simulink library "speedgoatlib_evse"  (R2024b)
settings: Solver=VariableStepAuto  StartTime=0.0  StopTime=10.0  RelTol=1e-3
undefined symbols (not defined in the file): sg_ev_charging_read_m, sg_ev_charging_write_m, sg_ev_isolation_read_m, sg_ev_parameter_read_m, sg_ev_parameter_write_m, sg_ev_precharge_read_m, sg_ev_precharge_write_m, sg_ev_status_m, sg_ev_stop_read_m, sg_ev_stop_write_m, sg_ev_welding_read_m, sg_ev_welding_write_m, sg_evse_charging_read_m, sg_evse_charging_write_m, sg_evse_isolation_read_m, sg_evse_isolation_write_m, sg_evse_parameter_read_m, sg_evse_parameter_write_m, sg_evse_precharge_read_m, sg_evse_precharge_write_m, sg_evse_status_m, sg_evse_stop_read_m, sg_evse_stop_write_m, sg_evse_welding_read_m, sg_evse_welding_write_m
libraries: speedgoatlib_mqtt x199, simulink x39, $bdroot x24
(part 3 of 8)

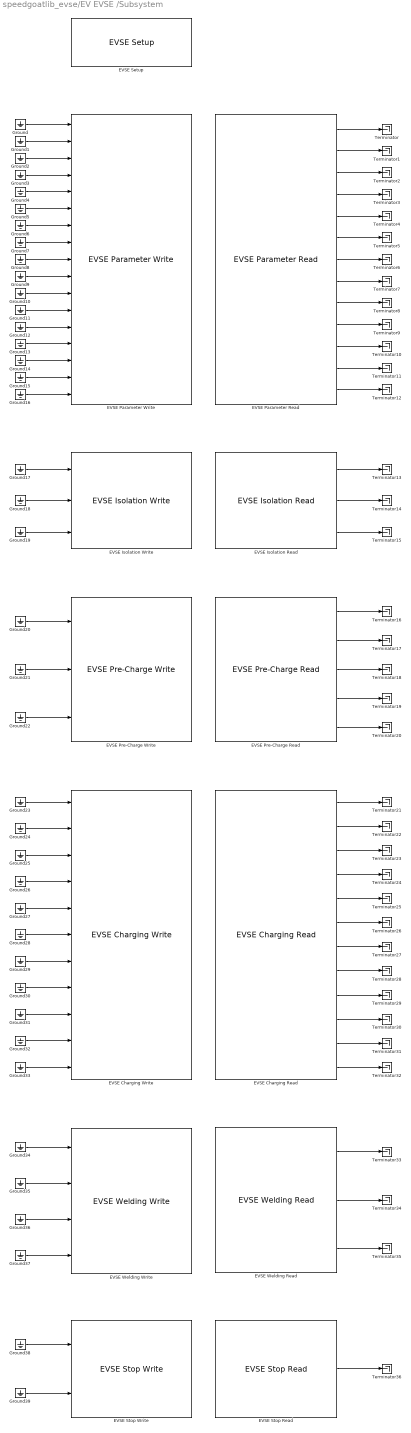
== system speedgoatlib_evse/EV EVSE /Subsystem ==
  "EVSE Charging Read " : $bdroot/Blocks by Charge State/EVSE Charging Read   parClientId=0  parConnectionId=0  parSampleTime=-1
  "EVSE Charging Write " : $bdroot/Blocks by Charge State/EVSE Charging Write   parClientId=0  parConnectionId=0  parSampleTime=-1  parEnNotification=off  parEnIsolationStatus=off  parEnStatusCode=off  parEnPresentVoltage=off  parEnPresentCurrent=off  parEnCurrentLimitAchieved=off  parEnVoltageLimitAchieved=off  parEnPowerLimitAchieved=off  parEnMaxVoltageLimit=off  parEnMaxCurrentLimit=off  parEnMaxPowerLimit=off
  "EVSE Isolation Read " : $bdroot/Blocks by Charge State/EVSE Isolation Read   parClientId=0  parConnectionId=0  parSampleTime=-1
  "EVSE Isolation Write " : $bdroot/Blocks by Charge State/EVSE Isolation Write   parClientId=0  parConnectionId=0  parSampleTime=-1  parEnEvseProcessing=off  parEnIsolationStatus=off  parEnStatusCode=off
  "EVSE Parameter Read " : $bdroot/Blocks by Charge State/EVSE Parameter Read   parClientId=0  parConnectionId=0  parSampleTime=-1
  "EVSE Parameter Write " : $bdroot/Blocks by Charge State/EVSE Parameter Write   parClientId=0  parConnectionId=0  parSampleTime=-1  parEnEvseProcessing=off  parEnSaScheduleList=off  parEnMaxVoltageLimit=off  parEnMaxCurrentLimit=off  parEnMaxPowerLimit=off  parEnMinVoltageLimit=off  parEnMinCurrentLimit=off  parEnCurrRegTol=off  parEnPeakCurrentRipple=off  parEnEnergyToBeDelivered=off  parEnNotificationMaxDelay=off  parEnNotification=off  parEnIsolationStatus=off  parEnStatusCode=off
  "EVSE Pre-Charge Read " : $bdroot/Blocks by Charge State/EVSE Pre-Charge Read   parClientId=0  parConnectionId=0  parSampleTime=-1
  "EVSE Pre-Charge Write " : $bdroot/Blocks by Charge State/EVSE Pre-Charge Write   parClientId=0  parConnectionId=0  parSampleTime=-1  parEnIsolationStatus=off  parEnStatusCode=off  parEnPresentVoltage=off
  "EVSE Setup " : $bdroot/Blocks by Charge State/EVSE Setup   parClientId=0  parConnectionId=0  parClientIdentifier='speedgoat'  parIpAddrStr='192.168.10.7'  parSampleTime=-1  parTcpPort=1883  parRemoteIpAddrStr='192.168.10.8'  parMaxVoltageLimit=480  parMaxCurrentLimit=100  parMinCurrentLimit=0  parMaxPowerLimit=60000  parMinVoltageLimit=12  parCurrRegTol=5  parPeakCurrentRipple=0
  "EVSE Stop Read " : $bdroot/Blocks by Charge State/EVSE Stop Read   parClientId=0  parConnectionId=0  parSampleTime=-1
  "EVSE Stop Write " : $bdroot/Blocks by Charge State/EVSE Stop Write   parClientId=0  parConnectionId=0  parSampleTime=-1  parEnStopProgress=off  parEnEvseProcessing=off
  "EVSE Welding Read " : $bdroot/Blocks by Charge State/EVSE Welding Read   parClientId=0  parConnectionId=0  parSampleTime=-1
  "EVSE Welding Write " : $bdroot/Blocks by Charge State/EVSE Welding Write   parClientId=0  parConnectionId=0  parSampleTime=-1  parEnNotification=off  parEnIsolationStatus=off  parEnStatusCode=off  parEnPresentVoltage=off
  Ground{,1..39} (40 alike) : Ground
  Terminator{,1..36} (37 alike) : Terminator
  wires:
  "EVSE Pre-Charge Read "/2 -> Terminator17/1
  Ground9/1 -> "EVSE Parameter Write "/10
  "EVSE Isolation Read "/2 -> Terminator14/1
  Ground17/1 -> "EVSE Isolation Write "/1
  Ground10/1 -> "EVSE Parameter Write "/11
  Ground14/1 -> "EVSE Parameter Write "/15
  Ground3/1 -> "EVSE Parameter Write "/4
  Ground11/1 -> "EVSE Parameter Write "/12
  "EVSE Parameter Read "/7 -> Terminator6/1
  "EVSE Parameter Read "/5 -> Terminator4/1
  "EVSE Parameter Read "/4 -> Terminator3/1
  Ground13/1 -> "EVSE Parameter Write "/14
  Ground5/1 -> "EVSE Parameter Write "/6
  "EVSE Parameter Read "/2 -> Terminator1/1
  Ground7/1 -> "EVSE Parameter Write "/8
  Ground6/1 -> "EVSE Parameter Write "/7
  Ground/1 -> "EVSE Parameter Write "/1
  Ground1/1 -> "EVSE Parameter Write "/2
  Ground30/1 -> "EVSE Charging Write "/8
  Ground8/1 -> "EVSE Parameter Write "/9
  "EVSE Charging Read "/9 -> Terminator29/1
  "EVSE Parameter Read "/8 -> Terminator7/1
  "EVSE Parameter Read "/10 -> Terminator9/1
  Ground19/1 -> "EVSE Isolation Write "/3
  "EVSE Parameter Read "/11 -> Terminator10/1
  "EVSE Pre-Charge Read "/4 -> Terminator19/1
  Ground31/1 -> "EVSE Charging Write "/9
  "EVSE Parameter Read "/9 -> Terminator8/1
  Ground23/1 -> "EVSE Charging Write "/1
  "EVSE Charging Read "/4 -> Terminator24/1
  Ground24/1 -> "EVSE Charging Write "/2
  "EVSE Charging Read "/2 -> Terminator22/1
  Ground33/1 -> "EVSE Charging Write "/11
  Ground2/1 -> "EVSE Parameter Write "/3
  Ground15/1 -> "EVSE Parameter Write "/16
  "EVSE Parameter Read "/12 -> Terminator11/1
  Ground18/1 -> "EVSE Isolation Write "/2
  Ground20/1 -> "EVSE Pre-Charge Write "/1
  "EVSE Stop Read "/1 -> Terminator36/1
  "EVSE Welding Read "/1 -> Terminator33/1
  "EVSE Pre-Charge Read "/1 -> Terminator16/1
  Ground39/1 -> "EVSE Stop Write "/2
  Ground16/1 -> "EVSE Parameter Write "/17
  Ground38/1 -> "EVSE Stop Write "/1
  Ground34/1 -> "EVSE Welding Write "/1
  "EVSE Welding Read "/3 -> Terminator35/1
  "EVSE Parameter Read "/1 -> Terminator/1
  Ground21/1 -> "EVSE Pre-Charge Write "/2
  Ground27/1 -> "EVSE Charging Write "/5
  Ground29/1 -> "EVSE Charging Write "/7
  "EVSE Isolation Read "/3 -> Terminator15/1
  "EVSE Welding Read "/2 -> Terminator34/1
  "EVSE Charging Read "/6 -> Terminator26/1
  "EVSE Charging Read "/7 -> Terminator27/1
  Ground4/1 -> "EVSE Parameter Write "/5
  Ground35/1 -> "EVSE Welding Write "/2
  "EVSE Charging Read "/3 -> Terminator23/1
  Ground22/1 -> "EVSE Pre-Charge Write "/3
  Ground12/1 -> "EVSE Parameter Write "/13
  "EVSE Charging Read "/1 -> Terminator21/1
  "EVSE Parameter Read "/3 -> Terminator2/1
  Ground26/1 -> "EVSE Charging Write "/4
  Ground37/1 -> "EVSE Welding Write "/4
  "EVSE Isolation Read "/1 -> Terminator13/1
  "EVSE Parameter Read "/13 -> Terminator12/1
  Ground36/1 -> "EVSE Welding Write "/3
  "EVSE Charging Read "/5 -> Terminator25/1
  Ground25/1 -> "EVSE Charging Write "/3
  Ground32/1 -> "EVSE Charging Write "/10
  "EVSE Charging Read "/8 -> Terminator28/1
  "EVSE Pre-Charge Read "/3 -> Terminator18/1
  "EVSE Charging Read "/12 -> Terminator32/1
  Ground28/1 -> "EVSE Charging Write "/6
  "EVSE Pre-Charge Read "/5 -> Terminator20/1
  "EVSE Charging Read "/10 -> Terminator30/1
  "EVSE Charging Read "/11 -> Terminator31/1
  "EVSE Parameter Read "/6 -> Terminator5/1

== system speedgoatlib_evse/EV Status /Authentication ==
  Auth Status Subscribe : speedgoatlib_mqtt/Client/MQTT Client Subscribe  ClientId=parClientId  ConnectionId=parConnectionId  Topic='port0/ci/charge/auth/status'  QoS=0 - at most once  InitValue=zeros(1,24,'uint8')  Extended=off  SampleTime=parSampleTime
      settings: SourceProductName=MQTT
  string compare logic : Subsystem
  Status : Outport
  wires:
  string compare logic/1(Output) -> Status/1
  Auth Status Subscribe/1 -> string compare logic/1(Input)

== system speedgoatlib_evse/EV Status /CP State ==
  ASCII to String1 : ASCIIToString
  Add : Sum  Inputs=++++++
  CP Status Subscribe : speedgoatlib_mqtt/Client/MQTT Client Subscribe  ClientId=parClientId  ConnectionId=parConnectionId  Topic='port0/ci/charge/cp/status'  QoS=0 - at most once  InitValue=zeros(1,24,'uint8')  Extended=off  SampleTime=parSampleTime
      settings: SourceProductName=MQTT
  Data Type Conversion{,1..5} (6 alike) : DataTypeConversion  OutDataTypeStr=double  SaturateOnIntegerOverflow=off  RndMeth=Floor
  Gain : Gain
  Gain1 : Gain  Gain=2
  Gain2 : Gain  Gain=3
  Gain3 : Gain  Gain=4
  Gain4 : Gain  Gain=5
  Gain5 : Gain  Gain=6
  String Compare{,1..5} (6 alike) : StringCompare  CaseSensitive=off
  String Constant : StringConstant  String="\"A\""
  String Constant1 : StringConstant  String="\"B\""
  String Constant2 : StringConstant  String="\"C\""
  String Constant3 : StringConstant  String="\"D\""
  String Constant4 : StringConstant  String="\"E\""
  String Constant5 : StringConstant  String="\"F\""
  CP State : Outport
  wires:
  Data Type Conversion5/1 -> Gain5/1
  Data Type Conversion4/1 -> Gain4/1
  Data Type Conversion3/1 -> Gain3/1
  Data Type Conversion2/1 -> Gain2/1
  Data Type Conversion1/1 -> Gain1/1
  Data Type Conversion/1 -> Gain/1
  Add/1 -> CP State/1
  Gain5/1 -> Add/6
  Gain4/1 -> Add/5
  Gain3/1 -> Add/4
  Gain2/1 -> Add/3
  Gain1/1 -> Add/2
  Gain/1 -> Add/1
  String Compare5/1 -> Data Type Conversion5/1
  String Compare4/1 -> Data Type Conversion4/1
  String Compare3/1 -> Data Type Conversion3/1
  String Compare2/1 -> Data Type Conversion2/1
  String Compare1/1 -> Data Type Conversion1/1
  String Compare/1 -> Data Type Conversion/1
  String Constant5/1 -> String Compare5/2
  String Constant4/1 -> String Compare4/2
  String Constant3/1 -> String Compare3/2
  String Constant2/1 -> String Compare2/2
  String Constant1/1 -> String Compare1/2
  CP Status Subscribe/1 -> ASCII to String1/1
  ASCII to String1/1 -> String Compare/1, String Compare1/1, String Compare2/1, String Compare3/1, String Compare4/1, String Compare5/1
  String Constant/1 -> String Compare/2

== system speedgoatlib_evse/EV Status /Charge ==
  Charge Status Subscribe : speedgoatlib_mqtt/Client/MQTT Client Subscribe  ClientId=parClientId  ConnectionId=parConnectionId  Topic='port0/ci/charge/charge/status'  QoS=0 - at most once  InitValue=zeros(1,24,'uint8')  Extended=off  SampleTime=parSampleTime
      settings: SourceProductName=MQTT
  string compare logic : Subsystem
  Status : Outport
  wires:
  string compare logic/1(Output) -> Status/1
  Charge Status Subscribe/1 -> string compare logic/1(Input)

== system speedgoatlib_evse/EV Status /Initialization ==
  Init Status Subscribe : speedgoatlib_mqtt/Client/MQTT Client Subscribe  ClientId=parClientId  ConnectionId=parConnectionId  Topic='port0/ci/charge/init/status'  QoS=0 - at most once  InitValue=zeros(1,24,'uint8')  Extended=off  SampleTime=parSampleTime
      settings: SourceProductName=MQTT
  string compare logic : Subsystem
  Status : Outport
  wires:
  string compare logic/1(Output) -> Status/1
  Init Status Subscribe/1 -> string compare logic/1(Input)

== system speedgoatlib_evse/EV Status /Isolation ==
  Isolation Status Subscribe : speedgoatlib_mqtt/Client/MQTT Client Subscribe  ClientId=parClientId  ConnectionId=parConnectionId  Topic='port0/ci/charge/isolation/status'  QoS=0 - at most once  InitValue=zeros(1,24,'uint8')  Extended=off  SampleTime=parSampleTime
      settings: SourceProductName=MQTT
  string compare logic : Subsystem
  Status : Outport
  wires:
  Isolation Status Subscribe/1 -> string compare logic/1(Input)
  string compare logic/1(Output) -> Status/1

== system speedgoatlib_evse/EV Status /PP State ==
  ASCII to String1 : ASCIIToString
  PP Status Subscribe : speedgoatlib_mqtt/Client/MQTT Client Subscribe  ClientId=parClientId  ConnectionId=parConnectionId  Topic='port0/ci/charge/pp/status'  QoS=0 - at most once  InitValue=zeros(1,8,'uint8')  Extended=off  SampleTime=parSampleTime
      settings: SourceProductName=MQTT
  String to Double6 : ScanString  Format="\"%lf\""
  PP State : Outport
  wires:
  String to Double6/1 -> PP State/1
  ASCII to String1/1 -> String to Double6/1
  PP Status Subscribe/1 -> ASCII to String1/1

== system speedgoatlib_evse/EV Status /PWM State ==
  ASCII to String1 : ASCIIToString
  PWM Status Subscribe : speedgoatlib_mqtt/Client/MQTT Client Subscribe  ClientId=parClientId  ConnectionId=parConnectionId  Topic='port0/ci/charge/pwm/status'  QoS=0 - at most once  InitValue=zeros(1,24,'uint8')  Extended=off  SampleTime=parSampleTime
      settings: SourceProductName=MQTT
  String to Double6 : ScanString  Format="\"%lf\""
  PP State : Outport
  wires:
  PWM Status Subscribe/1 -> ASCII to String1/1
  ASCII to String1/1 -> String to Double6/1
  String to Double6/1 -> PP State/1

== system speedgoatlib_evse/EV Status /Parameter ==
  Param Status Subscribe : speedgoatlib_mqtt/Client/MQTT Client Subscribe  ClientId=parClientId  ConnectionId=parConnectionId  Topic='port0/ci/charge/parameter/status'  QoS=0 - at most once  InitValue=zeros(1,24,'uint8')  Extended=off  SampleTime=parSampleTime
      settings: SourceProductName=MQTT
  string compare logic : Subsystem
  Status : Outport
  wires:
  Param Status Subscribe/1 -> string compare logic/1(Input)
  string compare logic/1(Output) -> Status/1

== system speedgoatlib_evse/EV Status /Plug State ==
  ASCII to String1 : ASCIIToString
  Add : Sum  Inputs=+++
  Data Type Conversion : DataTypeConversion  OutDataTypeStr=double  SaturateOnIntegerOverflow=off  RndMeth=Floor
  Data Type Conversion1 : DataTypeConversion  OutDataTypeStr=double  SaturateOnIntegerOverflow=off  RndMeth=Floor
  Data Type Conversion2 : DataTypeConversion  OutDataTypeStr=double  SaturateOnIntegerOverflow=off  RndMeth=Floor
  Gain : Gain  Gain=0
  Gain1 : Gain
  Gain2 : Gain  Gain=2
  Plug Status Subscribe : speedgoatlib_mqtt/Client/MQTT Client Subscribe  ClientId=parClientId  ConnectionId=parConnectionId  Topic='port0/ci/charge/plug/status'  QoS=0 - at most once  InitValue=zeros(1,24,'uint8')  Extended=off  SampleTime=parSampleTime
      settings: SourceProductName=Simulink Real-Time: Speedgoat I/O Blockset
  String Compare : StringCompare  CaseSensitive=off
  String Compare1 : StringCompare  CaseSensitive=off
  String Compare2 : StringCompare  CaseSensitive=off
  String Constant : StringConstant  String="\"unlocked\""
  String Constant1 : StringConstant  String="\"locked\""
  String Constant2 : StringConstant  String="\"unknown\""
  Plug State : Outport
  wires:
  Data Type Conversion2/1 -> Gain2/1
  Data Type Conversion1/1 -> Gain1/1
  Data Type Conversion/1 -> Gain/1
  Add/1 -> Plug State/1
  String Constant2/1 -> String Compare2/2
  Gain2/1 -> Add/3
  String Compare2/1 -> Data Type Conversion2/1
  Gain/1 -> Add/1
  String Compare1/1 -> Data Type Conversion1/1
  ASCII to String1/1 -> String Compare/1, String Compare1/1, String Compare2/1
  Gain1/1 -> Add/2
  Plug Status Subscribe/1 -> ASCII to String1/1
  String Constant/1 -> String Compare/2
  String Constant1/1 -> String Compare1/2
  String Compare/1 -> Data Type Conversion/1

== system speedgoatlib_evse/EV Status /Precharge ==
  Precharge Status Subscribe : speedgoatlib_mqtt/Client/MQTT Client Subscribe  ClientId=parClientId  ConnectionId=parConnectionId  Topic='port0/ci/charge/precharge/status'  QoS=0 - at most once  InitValue=zeros(1,24,'uint8')  Extended=off  SampleTime=parSampleTime
      settings: SourceProductName=MQTT
  string compare logic : Subsystem
  Status : Outport
  wires:
  string compare logic/1(Output) -> Status/1
  Precharge Status Subscribe/1 -> string compare logic/1(Input)

== system speedgoatlib_evse/EV Status /Selected Protocol ==
  ASCII to String1 : ASCIIToString
  Protocol Subscribe : speedgoatlib_mqtt/Client/MQTT Client Subscribe  ClientId=parClientId  ConnectionId=parConnectionId  Topic='port0/ci/charge/init/protocol'  QoS=0 - at most once  InitValue=zeros(1,24,'uint8')  Extended=off  SampleTime=parSampleTime
      settings: SourceProductName=MQTT
  Protocol : Outport
  wires:
  ASCII to String1/1 -> Protocol/1
  Protocol Subscribe/1 -> ASCII to String1/1

== system speedgoatlib_evse/EV Status /Stop ==
  Stop Status Subscribe : speedgoatlib_mqtt/Client/MQTT Client Subscribe  ClientId=parClientId  ConnectionId=parConnectionId  Topic='port0/ci/charge/stop/status'  QoS=0 - at most once  InitValue=zeros(1,24,'uint8')  Extended=off  SampleTime=parSampleTime
      settings: SourceProductName=MQTT
  string compare logic : Subsystem
  Status : Outport
  wires:
  string compare logic/1(Output) -> Status/1
  Stop Status Subscribe/1 -> string compare logic/1(Input)

== system speedgoatlib_evse/EV Status /TCP State ==
  ASCII to String1 : ASCIIToString
  String to Double6 : ScanString  Format="\"%lf\""
  TCP Status Subscribe : speedgoatlib_mqtt/Client/MQTT Client Subscribe  ClientId=parClientId  ConnectionId=parConnectionId  Topic='port0/ci/charge/tcp/status'  QoS=0 - at most once  InitValue=zeros(1,8,'uint8')  Extended=off  SampleTime=parSampleTime
      settings: SourceProductName=MQTT
  PP State : Outport
  wires:
  TCP Status Subscribe/1 -> ASCII to String1/1
  ASCII to String1/1 -> String to Double6/1
  String to Double6/1 -> PP State/1

== system speedgoatlib_evse/EV Status /Welding ==
  Welding Status Subscribe : speedgoatlib_mqtt/Client/MQTT Client Subscribe  ClientId=parClientId  ConnectionId=parConnectionId  Topic='port0/ci/charge/welding/status'  QoS=0 - at most once  InitValue=zeros(1,24,'uint8')  Extended=off  SampleTime=parSampleTime
      settings: SourceProductName=MQTT
  string compare logic : Subsystem
  Status : Outport
  wires:
  Welding Status Subscribe/1 -> string compare logic/1(Input)
  string compare logic/1(Output) -> Status/1

== system speedgoatlib_evse/EVSE Status /Authentication ==
  Auth Status Subscribe : speedgoatlib_mqtt/Client/MQTT Client Subscribe  ClientId=parClientId  ConnectionId=parConnectionId  Topic='port0/ci/charge/auth/status'  QoS=0 - at most once  InitValue=zeros(1,24,'uint8')  Extended=off  SampleTime=parSampleTime
      settings: SourceProductName=MQTT
  string compare logic : Subsystem
  Status : Outport
  wires:
  Auth Status Subscribe/1 -> string compare logic/1(Input)
  string compare logic/1(Output) -> Status/1

== system speedgoatlib_evse/EVSE Status /CP State ==
  ASCII to String1 : ASCIIToString
  Add : Sum  Inputs=++++++
  CP Status Subscribe : speedgoatlib_mqtt/Client/MQTT Client Subscribe  ClientId=parClientId  ConnectionId=parConnectionId  Topic='port0/ci/charge/cp/status'  QoS=0 - at most once  InitValue=zeros(1,24,'uint8')  Extended=off  SampleTime=parSampleTime
      settings: SourceProductName=MQTT
  Data Type Conversion{,1..5} (6 alike) : DataTypeConversion  OutDataTypeStr=double  SaturateOnIntegerOverflow=off  RndMeth=Floor
  Gain : Gain
  Gain1 : Gain  Gain=2
  Gain2 : Gain  Gain=3
  Gain3 : Gain  Gain=4
  Gain4 : Gain  Gain=5
  Gain5 : Gain  Gain=6
  String Compare{,1..5} (6 alike) : StringCompare  CaseSensitive=off
  String Constant : StringConstant  String="\"A\""
  String Constant1 : StringConstant  String="\"B\""
  String Constant2 : StringConstant  String="\"C\""
  String Constant3 : StringConstant  String="\"D\""
  String Constant4 : StringConstant  String="\"E\""
  String Constant5 : StringConstant  String="\"F\""
  CP State : Outport
  wires:
  String Constant/1 -> String Compare/2
  ASCII to String1/1 -> String Compare5/1, String Compare4/1, String Compare3/1, String Compare2/1, String Compare1/1, String Compare/1
  CP Status Subscribe/1 -> ASCII to String1/1
  String Constant1/1 -> String Compare1/2
  String Constant2/1 -> String Compare2/2
  String Constant3/1 -> String Compare3/2
  String Constant4/1 -> String Compare4/2
  String Constant5/1 -> String Compare5/2
  String Compare/1 -> Data Type Conversion/1
  String Compare1/1 -> Data Type Conversion1/1
  String Compare2/1 -> Data Type Conversion2/1
  String Compare3/1 -> Data Type Conversion3/1
  String Compare4/1 -> Data Type Conversion4/1
  String Compare5/1 -> Data Type Conversion5/1
  Gain/1 -> Add/1
  Gain1/1 -> Add/2
  Gain2/1 -> Add/3
  Gain3/1 -> Add/4
  Gain4/1 -> Add/5
  Gain5/1 -> Add/6
  Add/1 -> CP State/1
  Data Type Conversion/1 -> Gain/1
  Data Type Conversion1/1 -> Gain1/1
  Data Type Conversion2/1 -> Gain2/1
  Data Type Conversion3/1 -> Gain3/1
  Data Type Conversion4/1 -> Gain4/1
  Data Type Conversion5/1 -> Gain5/1

== system speedgoatlib_evse/EVSE Status /Charge ==
  Charge Status Subscribe : speedgoatlib_mqtt/Client/MQTT Client Subscribe  ClientId=parClientId  ConnectionId=parConnectionId  Topic='port0/ci/charge/charge/status'  QoS=0 - at most once  InitValue=zeros(1,24,'uint8')  Extended=off  SampleTime=parSampleTime
      settings: SourceProductName=MQTT
  string compare logic : Subsystem
  Status : Outport
  wires:
  Charge Status Subscribe/1 -> string compare logic/1(Input)
  string compare logic/1(Output) -> Status/1

== system speedgoatlib_evse/EVSE Status /Initialization ==
  Init Status Subscribe : speedgoatlib_mqtt/Client/MQTT Client Subscribe  ClientId=parClientId  ConnectionId=parConnectionId  Topic='port0/ci/charge/init/status'  QoS=0 - at most once  InitValue=zeros(1,24,'uint8')  Extended=off  SampleTime=parSampleTime
      settings: SourceProductName=MQTT
  string compare logic : Subsystem
  Status : Outport
  wires:
  Init Status Subscribe/1 -> string compare logic/1(Input)
  string compare logic/1(Output) -> Status/1

== system speedgoatlib_evse/EVSE Status /Isolation ==
  Isolation Status Subscribe : speedgoatlib_mqtt/Client/MQTT Client Subscribe  ClientId=parClientId  ConnectionId=parConnectionId  Topic='port0/ci/charge/isolation/status'  QoS=0 - at most once  InitValue=zeros(1,24,'uint8')  Extended=off  SampleTime=parSampleTime
      settings: SourceProductName=MQTT
  string compare logic : Subsystem
  Status : Outport
  wires:
  string compare logic/1(Output) -> Status/1
  Isolation Status Subscribe/1 -> string compare logic/1(Input)

== system speedgoatlib_evse/EVSE Status /PP State ==
  ASCII to String1 : ASCIIToString
  PP Status Subscribe : speedgoatlib_mqtt/Client/MQTT Client Subscribe  ClientId=parClientId  ConnectionId=parConnectionId  Topic='port0/ci/charge/pp/status'  QoS=0 - at most once  InitValue=zeros(1,8,'uint8')  Extended=off  SampleTime=parSampleTime
      settings: SourceProductName=MQTT
  String to Double6 : ScanString  Format="\"%lf\""
  PP State : Outport
  wires:
  PP Status Subscribe/1 -> ASCII to String1/1
  ASCII to String1/1 -> String to Double6/1
  String to Double6/1 -> PP State/1

== system speedgoatlib_evse/EVSE Status /PWM State ==
  ASCII to String1 : ASCIIToString
  PWM Status Subscribe : speedgoatlib_mqtt/Client/MQTT Client Subscribe  ClientId=parClientId  ConnectionId=parConnectionId  Topic='port0/ci/charge/pwm/status'  QoS=0 - at most once  InitValue=zeros(1,24,'uint8')  Extended=off  SampleTime=parSampleTime
      settings: SourceProductName=MQTT
  String to Double6 : ScanString  Format="\"%lf\""
  PP State : Outport
  wires:
  String to Double6/1 -> PP State/1
  ASCII to String1/1 -> String to Double6/1
  PWM Status Subscribe/1 -> ASCII to String1/1

== system speedgoatlib_evse/EVSE Status /Parameter ==
  Param Status Subscribe : speedgoatlib_mqtt/Client/MQTT Client Subscribe  ClientId=parClientId  ConnectionId=parConnectionId  Topic='port0/ci/charge/parameter/status'  QoS=0 - at most once  InitValue=zeros(1,24,'uint8')  Extended=off  SampleTime=parSampleTime
      settings: SourceProductName=MQTT
  string compare logic : Subsystem
  Status : Outport
  wires:
  string compare logic/1(Output) -> Status/1
  Param Status Subscribe/1 -> string compare logic/1(Input)

== system speedgoatlib_evse/EVSE Status /Plug State ==
  ASCII to String1 : ASCIIToString
  Add : Sum  Inputs=+++
  Data Type Conversion : DataTypeConversion  OutDataTypeStr=double  SaturateOnIntegerOverflow=off  RndMeth=Floor
  Data Type Conversion1 : DataTypeConversion  OutDataTypeStr=double  SaturateOnIntegerOverflow=off  RndMeth=Floor
  Data Type Conversion2 : DataTypeConversion  OutDataTypeStr=double  SaturateOnIntegerOverflow=off  RndMeth=Floor
  Gain : Gain  Gain=0
  Gain1 : Gain
  Gain2 : Gain  Gain=2
  Plug Status Subscribe : speedgoatlib_mqtt/Client/MQTT Client Subscribe  ClientId=parClientId  ConnectionId=parConnectionId  Topic='port0/ci/charge/plug/status'  QoS=0 - at most once  InitValue=zeros(1,24,'uint8')  Extended=off  SampleTime=parSampleTime
      settings: SourceProductName=MQTT
  String Compare : StringCompare  CaseSensitive=off
  String Compare1 : StringCompare  CaseSensitive=off
  String Compare2 : StringCompare  CaseSensitive=off
  String Constant : StringConstant  String="\"unlocked\""
  String Constant1 : StringConstant  String="\"locked\""
  String Constant2 : StringConstant  String="\"unknown\""
  Plug State : Outport
  wires:
  String Compare/1 -> Data Type Conversion/1
  String Constant1/1 -> String Compare1/2
  String Constant/1 -> String Compare/2
  Plug Status Subscribe/1 -> ASCII to String1/1
  Gain1/1 -> Add/2
  ASCII to String1/1 -> String Compare2/1, String Compare1/1, String Compare/1
  String Compare1/1 -> Data Type Conversion1/1
  Gain/1 -> Add/1
  String Compare2/1 -> Data Type Conversion2/1
  Gain2/1 -> Add/3
  String Constant2/1 -> String Compare2/2
  Add/1 -> Plug State/1
  Data Type Conversion/1 -> Gain/1
  Data Type Conversion1/1 -> Gain1/1
  Data Type Conversion2/1 -> Gain2/1

== system speedgoatlib_evse/EVSE Status /Precharge ==
  Precharge Status Subscribe : speedgoatlib_mqtt/Client/MQTT Client Subscribe  ClientId=parClientId  ConnectionId=parConnectionId  Topic='port0/ci/charge/precharge/status'  QoS=0 - at most once  InitValue=zeros(1,24,'uint8')  Extended=off  SampleTime=parSampleTime
      settings: SourceProductName=MQTT
  string compare logic : Subsystem
  Status : Outport
  wires:
  Precharge Status Subscribe/1 -> string compare logic/1(Input)
  string compare logic/1(Output) -> Status/1

== system speedgoatlib_evse/EVSE Status /Selected Protocol ==
  ASCII to String1 : ASCIIToString
  Protocol Subscribe : speedgoatlib_mqtt/Client/MQTT Client Subscribe  ClientId=parClientId  ConnectionId=parConnectionId  Topic='port0/ci/charge/init/protocol'  QoS=0 - at most once  InitValue=zeros(1,24,'uint8')  Extended=off  SampleTime=parSampleTime
      settings: SourceProductName=MQTT
  Protocol : Outport
  wires:
  Protocol Subscribe/1 -> ASCII to String1/1
  ASCII to String1/1 -> Protocol/1

== system speedgoatlib_evse/EVSE Status /Stop ==
  Stop Status Subscribe : speedgoatlib_mqtt/Client/MQTT Client Subscribe  ClientId=parClientId  ConnectionId=parConnectionId  Topic='port0/ci/charge/stop/status'  QoS=0 - at most once  InitValue=zeros(1,24,'uint8')  Extended=off  SampleTime=parSampleTime
      settings: SourceProductName=MQTT
  string compare logic : Subsystem
  Status : Outport
  wires:
  Stop Status Subscribe/1 -> string compare logic/1(Input)
  string compare logic/1(Output) -> Status/1

== system speedgoatlib_evse/EVSE Status /TCP State ==
  ASCII to String1 : ASCIIToString
  String to Double6 : ScanString  Format="\"%lf\""
  TCP Status Subscribe : speedgoatlib_mqtt/Client/MQTT Client Subscribe  ClientId=parClientId  ConnectionId=parConnectionId  Topic='port0/ci/charge/tcp/status'  QoS=0 - at most once  InitValue=zeros(1,8,'uint8')  Extended=off  SampleTime=parSampleTime
      settings: SourceProductName=MQTT
  PP State : Outport
  wires:
  String to Double6/1 -> PP State/1
  ASCII to String1/1 -> String to Double6/1
  TCP Status Subscribe/1 -> ASCII to String1/1

== system speedgoatlib_evse/EVSE Status /Welding ==
  Welding Status Subscribe : speedgoatlib_mqtt/Client/MQTT Client Subscribe  ClientId=parClientId  ConnectionId=parConnectionId  Topic='port0/ci/charge/welding/status'  QoS=0 - at most once  InitValue=zeros(1,24,'uint8')  Extended=off  SampleTime=parSampleTime
      settings: SourceProductName=MQTT
  string compare logic : Subsystem
  Status : Outport
  wires:
  string compare logic/1(Output) -> Status/1
  Welding Status Subscribe/1 -> string compare logic/1(Input)

== system speedgoatlib_evse/Blocks by Charge State/EV Charging Read /Enabled Subsystem ==
  Enable : EnablePort
  ASCII to String1 : ASCIIToString
  ASCII to String2 : ASCIIToString
  ASCII to String5 : ASCIIToString
  Data Type Conversion3 : DataTypeConversion  OutDataTypeStr=boolean  SaturateOnIntegerOverflow=off  RndMeth=Floor
  Data Type Conversion4 : DataTypeConversion  OutDataTypeStr=boolean  SaturateOnIntegerOverflow=off  RndMeth=Floor
  Data Type Conversion5 : DataTypeConversion  OutDataTypeStr=boolean  SaturateOnIntegerOverflow=off  RndMeth=Floor
  Function Caller{,1..4} (5 alike) : FunctionCaller  FunctionPrototype=value = fromJsonPhysicalValue(uint8_vec)  InputArgumentSpecifications=zeros(1,48,'uint8')  OutputArgumentSpecifications=double(0)
  Simulink Function : Subsystem  TreatAsAtomicUnit=on
  String to Double : ScanString  Format="\"%lf\""
  String to Double1 : ScanString  Format="\"%lf\""
  String to Double2 : ScanString  Format="\"%lf\""
  port0_ci_evse_charge_currentlimitachieved : S-Function  FunctionName=sg_mqtt_client_subscribe_s  Parameters="ClientId,  ConnectionId, Topic, QoS, InitValue, Extended, SampleTime"  SFunctionDeploymentMode=off  EnableBusSupport=off  mask(mqtt_client_subscribe_1){ClientId=parClientId, ConnectionId=parConnectionId, Topic='port0/ci/evse/charge/currentlimitachieved', QoS=0 - at most once, InitValue=zeros(1,8,'uint8'), Extended=off, SampleTime=parSampleTime}
      mask prompts: ClientId "Station ID"; ConnectionId "Connection ID"; QoS "Quality of Service"; InitValue "Init Value"; Extended "Extended Interface"; SampleTime "Sample Time [s]"
      mask help: Speedgoat Driver Block<br>MQTT Client - Subscribe<br><br>&copy; 2007 - 2023, Speedgoat GmbH, <a href="matlab: web('www.speedgoat.com','-browser');">www.speedgoat.com</a>
      mask init:
      | sg_mqtt_client_subscribe_m.runMaskInitialization(ClientId, ConnectionId, Topic, InitValue, Extended);
      mask Help: eval('sg.utils.help.show(''io_main/refentry_mqtt_client_subscribe'');')
      mask TypeOptions QoS: 0 - at most once | 1 - at least once | 2 - exactly once
      mask DialogControl groupParameters Prompt: Parameters
      mask Display: disp('Speedgoat\nMQTT Client\nSubscribe\nStation ID: 0\nConnection ID: 0');
  port0_ci_evse_charge_maxcurrentlimit : S-Function  FunctionName=sg_mqtt_client_subscribe_s  Parameters="ClientId,  ConnectionId, Topic, QoS, InitValue, Extended, SampleTime"  SFunctionDeploymentMode=off  EnableBusSupport=off  mask(mqtt_client_subscribe_1){ClientId=parClientId, ConnectionId=parConnectionId, Topic='port0/ci/evse/charge/maxcurrentlimit', QoS=0 - at most once, InitValue=zeros(1,48,'uint8'), Extended=off, SampleTime=parSampleTime}
      mask prompts: ClientId "Station ID"; ConnectionId "Connection ID"; QoS "Quality of Service"; InitValue "Init Value"; Extended "Extended Interface"; SampleTime "Sample Time [s]"
      mask help: Speedgoat Driver Block<br>MQTT Client - Subscribe<br><br>&copy; 2007 - 2023, Speedgoat GmbH, <a href="matlab: web('www.speedgoat.com','-browser');">www.speedgoat.com</a>
      mask init:
      | sg_mqtt_client_subscribe_m.runMaskInitialization(ClientId, ConnectionId, Topic, InitValue, Extended);
      mask Help: eval('sg.utils.help.show(''io_main/refentry_mqtt_client_subscribe'');')
      mask TypeOptions QoS: 0 - at most once | 1 - at least once | 2 - exactly once
      mask DialogControl groupParameters Prompt: Parameters
      mask Display: disp('Speedgoat\nMQTT Client\nSubscribe\nStation ID: 0\nConnection ID: 0');
  port0_ci_evse_charge_maxpowerlimit : S-Function  FunctionName=sg_mqtt_client_subscribe_s  Parameters="ClientId,  ConnectionId, Topic, QoS, InitValue, Extended, SampleTime"  SFunctionDeploymentMode=off  EnableBusSupport=off  mask(mqtt_client_subscribe_1){ClientId=parClientId, ConnectionId=parConnectionId, Topic='port0/ci/evse/charge/maxpowerlimit', QoS=0 - at most once, InitValue=zeros(1,48,'uint8'), Extended=off, SampleTime=parSampleTime}
      mask prompts: ClientId "Station ID"; ConnectionId "Connection ID"; QoS "Quality of Service"; InitValue "Init Value"; Extended "Extended Interface"; SampleTime "Sample Time [s]"
      mask help: Speedgoat Driver Block<br>MQTT Client - Subscribe<br><br>&copy; 2007 - 2023, Speedgoat GmbH, <a href="matlab: web('www.speedgoat.com','-browser');">www.speedgoat.com</a>
      mask init:
      | sg_mqtt_client_subscribe_m.runMaskInitialization(ClientId, ConnectionId, Topic, InitValue, Extended);
      mask Help: eval('sg.utils.help.show(''io_main/refentry_mqtt_client_subscribe'');')
      mask TypeOptions QoS: 0 - at most once | 1 - at least once | 2 - exactly once
      mask DialogControl groupParameters Prompt: Parameters
      mask Display: disp('Speedgoat\nMQTT Client\nSubscribe\nStation ID: 0\nConnection ID: 0');
  port0_ci_evse_charge_maxvoltagelimit : speedgoatlib_mqtt/Client/MQTT Client Subscribe  ClientId=parClientId  ConnectionId=parConnectionId  Topic='port0/ci/evse/charge/maxvoltagelimit'  QoS=0 - at most once  InitValue=zeros(1,48,'uint8')  Extended=off  SampleTime=parSampleTime
      settings: SourceProductName=MQTT
  port0_ci_evse_charge_powerlimitachieved : S-Function  FunctionName=sg_mqtt_client_subscribe_s  Parameters="ClientId,  ConnectionId, Topic, QoS, InitValue, Extended, SampleTime"  SFunctionDeploymentMode=off  EnableBusSupport=off  mask(mqtt_client_subscribe_1){ClientId=parClientId, ConnectionId=parConnectionId, Topic='port0/ci/evse/charge/powerlimitachieved', QoS=0 - at most once, InitValue=zeros(1,8,'uint8'), Extended=off, SampleTime=parSampleTime}
      mask prompts: ClientId "Station ID"; ConnectionId "Connection ID"; QoS "Quality of Service"; InitValue "Init Value"; Extended "Extended Interface"; SampleTime "Sample Time [s]"
      mask help: Speedgoat Driver Block<br>MQTT Client - Subscribe<br><br>&copy; 2007 - 2023, Speedgoat GmbH, <a href="matlab: web('www.speedgoat.com','-browser');">www.speedgoat.com</a>
      mask init:
      | sg_mqtt_client_subscribe_m.runMaskInitialization(ClientId, ConnectionId, Topic, InitValue, Extended);
      mask Help: eval('sg.utils.help.show(''io_main/refentry_mqtt_client_subscribe'');')
      mask TypeOptions QoS: 0 - at most once | 1 - at least once | 2 - exactly once
      mask DialogControl groupParameters Prompt: Parameters
      mask Display: disp('Speedgoat\nMQTT Client\nSubscribe\nStation ID: 0\nConnection ID: 0');
  port0_ci_evse_charge_presentcurrent : S-Function  FunctionName=sg_mqtt_client_subscribe_s  Parameters="ClientId,  ConnectionId, Topic, QoS, InitValue, Extended, SampleTime"  SFunctionDeploymentMode=off  EnableBusSupport=off  mask(mqtt_client_subscribe_1){ClientId=parClientId, ConnectionId=parConnectionId, Topic='port0/ci/evse/charge/presentcurrent', QoS=0 - at most once, InitValue=zeros(1,48,'uint8'), Extended=off, SampleTime=parSampleTime}
      mask prompts: ClientId "Station ID"; ConnectionId "Connection ID"; QoS "Quality of Service"; InitValue "Init Value"; Extended "Extended Interface"; SampleTime "Sample Time [s]"
      mask help: Speedgoat Driver Block<br>MQTT Client - Subscribe<br><br>&copy; 2007 - 2023, Speedgoat GmbH, <a href="matlab: web('www.speedgoat.com','-browser');">www.speedgoat.com</a>
      mask init:
      | sg_mqtt_client_subscribe_m.runMaskInitialization(ClientId, ConnectionId, Topic, InitValue, Extended);
      mask Help: eval('sg.utils.help.show(''io_main/refentry_mqtt_client_subscribe'');')
      mask TypeOptions QoS: 0 - at most once | 1 - at least once | 2 - exactly once
      mask DialogControl groupParameters Prompt: Parameters
      mask Display: disp('Speedgoat\nMQTT Client\nSubscribe\nStation ID: 0\nConnection ID: 0');
  port0_ci_evse_charge_presentvoltage : S-Function  FunctionName=sg_mqtt_client_subscribe_s  Parameters="ClientId,  ConnectionId, Topic, QoS, InitValue, Extended, SampleTime"  SFunctionDeploymentMode=off  EnableBusSupport=off  mask(mqtt_client_subscribe_1){ClientId=parClientId, ConnectionId=parConnectionId, Topic='port0/ci/evse/charge/presentvoltage', QoS=0 - at most once, InitValue=zeros(1,48,'uint8'), Extended=off, SampleTime=parSampleTime}
      mask prompts: ClientId "Station ID"; ConnectionId "Connection ID"; QoS "Quality of Service"; InitValue "Init Value"; Extended "Extended Interface"; SampleTime "Sample Time [s]"
      mask help: Speedgoat Driver Block<br>MQTT Client - Subscribe<br><br>&copy; 2007 - 2023, Speedgoat GmbH, <a href="matlab: web('www.speedgoat.com','-browser');">www.speedgoat.com</a>
      mask init:
      | sg_mqtt_client_subscribe_m.runMaskInitialization(ClientId, ConnectionId, Topic, InitValue, Extended);
      mask Help: eval('sg.utils.help.show(''io_main/refentry_mqtt_client_subscribe'');')
      mask TypeOptions QoS: 0 - at most once | 1 - at least once | 2 - exactly once
      mask DialogControl groupParameters Prompt: Parameters
      mask Display: disp('Speedgoat\nMQTT Client\nSubscribe\nStation ID: 0\nConnection ID: 0');
  port0_ci_evse_charge_voltagelimitachieved : S-Function  FunctionName=sg_mqtt_client_subscribe_s  Parameters="ClientId,  ConnectionId, Topic, QoS, InitValue, Extended, SampleTime"  SFunctionDeploymentMode=off  EnableBusSupport=off  mask(mqtt_client_subscribe_1){ClientId=parClientId, ConnectionId=parConnectionId, Topic='port0/ci/evse/charge/voltagelimitachieved', QoS=0 - at most once, InitValue=zeros(1,8,'uint8'), Extended=off, SampleTime=parSampleTime}
      mask prompts: ClientId "Station ID"; ConnectionId "Connection ID"; QoS "Quality of Service"; InitValue "Init Value"; Extended "Extended Interface"; SampleTime "Sample Time [s]"
      mask help: Speedgoat Driver Block<br>MQTT Client - Subscribe<br><br>&copy; 2007 - 2023, Speedgoat GmbH, <a href="matlab: web('www.speedgoat.com','-browser');">www.speedgoat.com</a>
      mask init:
      | sg_mqtt_client_subscribe_m.runMaskInitialization(ClientId, ConnectionId, Topic, InitValue, Extended);
      mask Help: eval('sg.utils.help.show(''io_main/refentry_mqtt_client_subscribe'');')
      mask TypeOptions QoS: 0 - at most once | 1 - at least once | 2 - exactly once
      mask DialogControl groupParameters Prompt: Parameters
      mask Display: disp('Speedgoat\nMQTT Client\nSubscribe\nStation ID: 0\nConnection ID: 0');
  EVSE Present Voltage : Outport
  EVSE Present Current : Outport  Port=2
  EVSE Current Limit Achieved : Outport  Port=3
  EVSE Voltage Limit Achieved : Outport  Port=4
  EVSE Power Limit Achieved : Outport  Port=5
  EVSE Max Voltage Limit : Outport  Port=6
  EVSE Max Current Limit : Outport  Port=7
  EVSE Max Power Limit : Outport  Port=8
  wires:
  Function Caller4/1 -> EVSE Max Power Limit/1
  port0_ci_evse_charge_maxpowerlimit/1 -> Function Caller4/1
  port0_ci_evse_charge_maxcurrentlimit/1 -> Function Caller3/1
  Function Caller3/1 -> EVSE Max Current Limit/1
  Function Caller2/1 -> EVSE Max Voltage Limit/1
  port0_ci_evse_charge_maxvoltagelimit/1 -> Function Caller2/1
  Data Type Conversion4/1 -> EVSE Voltage Limit Achieved/1
  port0_ci_evse_charge_voltagelimitachieved/1 -> ASCII to String2/1
  port0_ci_evse_charge_currentlimitachieved/1 -> ASCII to String1/1
  Data Type Conversion3/1 -> EVSE Current Limit Achieved/1
  Function Caller1/1 -> EVSE Present Current/1
  port0_ci_evse_charge_presentcurrent/1 -> Function Caller1/1
  port0_ci_evse_charge_presentvoltage/1 -> Function Caller/1
  Function Caller/1 -> EVSE Present Voltage/1
  String to Double/1 -> Data Type Conversion3/1
  ASCII to String1/1 -> String to Double/1
  ASCII to String2/1 -> String to Double1/1
  String to Double1/1 -> Data Type Conversion4/1
  port0_ci_evse_charge_powerlimitachieved/1 -> ASCII to String5/1
  String to Double2/1 -> Data Type Conversion5/1
  Data Type Conversion5/1 -> EVSE Power Limit Achieved/1
  ASCII to String5/1 -> String to Double2/1

== system speedgoatlib_evse/Blocks by Charge State/EV Charging Read /string compare logic1 ==
  Input : Inport
  ASCII to String1 : ASCIIToString
  Add : Sum
  Gain : Gain  Gain=2
  String Compare : StringCompare
  String Compare1 : StringCompare
  String Constant : StringConstant  String="\"started\""
  String Constant1 : StringConstant  String="\"finished\""
  Out1 : Outport
  wires:
  ASCII to String1/1 -> String Compare1/1, String Compare/1
  String Constant1/1 -> String Compare1/2
  String Compare/1 -> Add/1
  String Constant/1 -> String Compare/2
  String Compare1/1 -> Gain/1
  Gain/1 -> Add/2
  Add/1 -> Out1/1
  Input/1 -> ASCII to String1/1

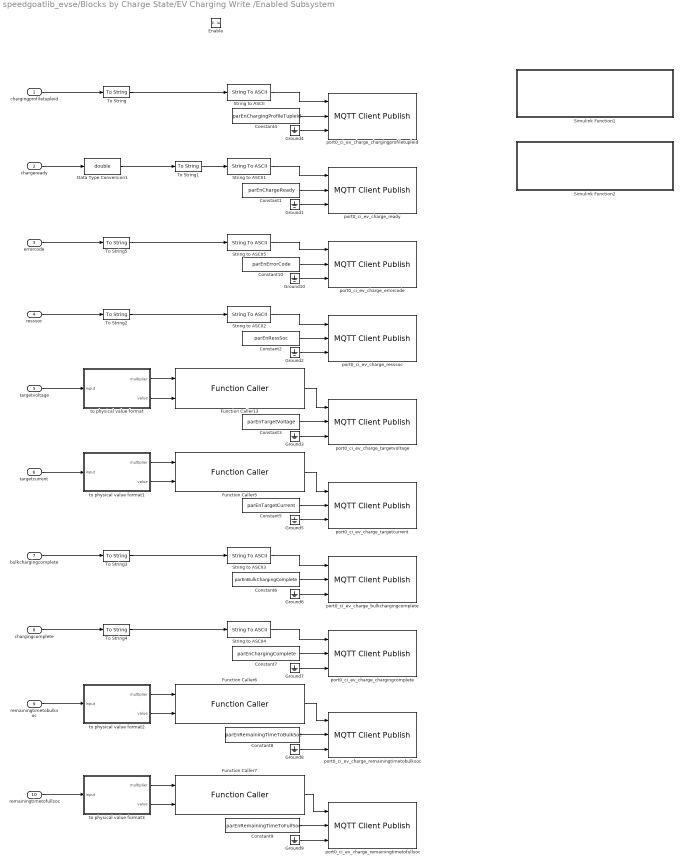
== system speedgoatlib_evse/Blocks by Charge State/EV Charging Write /Enabled Subsystem ==
  chargingprofiletupleid : Inport
  chargeready : Inport  Port=2
  errorcode : Inport  Port=3
  resssoc : Inport  Port=4
  targetvoltage : Inport  Port=5
  targetcurrent : Inport  Port=6
  bulkchargingcomplete : Inport  Port=7
  chargingcomplete : Inport  Port=8
  remainingtimetobulksoc : Inport  Port=9
  remainingtimetofullsoc : Inport  Port=10
  Enable : EnablePort
  Constant1 : Constant  Value=parEnChargeReady  OutDataTypeStr=boolean
  Constant10 : Constant  Value=parEnErrorCode  OutDataTypeStr=boolean
  Constant2 : Constant  Value=parEnRessSoc  OutDataTypeStr=boolean
  Constant3 : Constant  Value=parEnTargetVoltage  OutDataTypeStr=boolean
  Constant4 : Constant  Value=parEnChargingProfileTupleId  OutDataTypeStr=boolean
  Constant5 : Constant  Value=parEnTargetCurrent  OutDataTypeStr=boolean
  Constant6 : Constant  Value=parEnBulkChargingComplete  OutDataTypeStr=boolean
  Constant7 : Constant  Value=parEnChargingComplete  OutDataTypeStr=boolean
  Constant8 : Constant  Value=parEnRemainingTimeToBulkSoc  OutDataTypeStr=boolean
  Constant9 : Constant  Value=parEnRemainingTimeToFullSoc  OutDataTypeStr=boolean
  Data Type Conversion1 : DataTypeConversion  OutDataTypeStr=double  SaturateOnIntegerOverflow=off  RndMeth=Floor
  Function Caller13 : FunctionCaller  FunctionPrototype=json_string = toJsonPhysicalValue(multiplier,value)  InputArgumentSpecifications=double(0), double(0)  OutputArgumentSpecifications=zeros(1,48,'uint8')
  Function Caller5 : FunctionCaller  FunctionPrototype=json_string = toJsonPhysicalValue(multiplier,value)  InputArgumentSpecifications=double(0), double(0)  OutputArgumentSpecifications=zeros(1,48,'uint8')
  Function Caller6 : FunctionCaller  FunctionPrototype=json_string = toJsonPhysicalValueWithUnit(multiplier,value)  InputArgumentSpecifications=double(0), double(0)  OutputArgumentSpecifications=zeros(1,64,'uint8')
  Function Caller7 : FunctionCaller  FunctionPrototype=json_string = toJsonPhysicalValueWithUnit(multiplier,value)  InputArgumentSpecifications=double(0), double(0)  OutputArgumentSpecifications=zeros(1,64,'uint8')
  Ground{1..10} (10 alike) : Ground
  Simulink Function1 : Subsystem  TreatAsAtomicUnit=on
  Simulink Function2 : Subsystem  TreatAsAtomicUnit=on
  String to ASCII{,1..4} (5 alike) : StringToASCII  OutputVectorSize=12
  String to ASCII5 : StringToASCII  OutputVectorSize=24
  To String{,1..5} (6 alike) : ToString
  port0_ci_ev_charge_bulkchargingcomplete : speedgoatlib_mqtt/Client/MQTT Client Publish  ClientId=parClientId  ConnectionId=parConnectionId  Topic='port0/ci/ev/charge/bulkchargingcomplete'  QoS=0 - at most once  Retain=on  Extended=on  SampleTime=parSampleTime
      settings: SourceProductName=MQTT
  port0_ci_ev_charge_chargingcomplete : speedgoatlib_mqtt/Client/MQTT Client Publish  ClientId=parClientId  ConnectionId=parConnectionId  Topic='port0/ci/ev/charge/chargingcomplete'  QoS=0 - at most once  Retain=on  Extended=on  SampleTime=parSampleTime
      settings: SourceProductName=MQTT
  port0_ci_ev_charge_chargingprofiletupleid : speedgoatlib_mqtt/Client/MQTT Client Publish  ClientId=parClientId  ConnectionId=parConnectionId  Topic='port0/ci/ev/charge/chargingprofiletupleid'  QoS=0 - at most once  Retain=on  Extended=on  SampleTime=parSampleTime
      settings: SourceProductName=MQTT
  port0_ci_ev_charge_errorcode : speedgoatlib_mqtt/Client/MQTT Client Publish  ClientId=parClientId  ConnectionId=parConnectionId  Topic='port0/ci/ev/charge/errorcode'  QoS=0 - at most once  Retain=on  Extended=on  SampleTime=parSampleTime
      settings: SourceProductName=MQTT
  port0_ci_ev_charge_ready : speedgoatlib_mqtt/Client/MQTT Client Publish  ClientId=parClientId  ConnectionId=parConnectionId  Topic='port0/ci/ev/charge/ready'  QoS=0 - at most once  Retain=on  Extended=on  SampleTime=parSampleTime
      settings: SourceProductName=MQTT
  port0_ci_ev_charge_remainingtimetobulksoc : speedgoatlib_mqtt/Client/MQTT Client Publish  ClientId=parClientId  ConnectionId=parConnectionId  Topic='port0/ci/ev/charge/remainingtimetobulksoc'  QoS=0 - at most once  Retain=on  Extended=on  SampleTime=parSampleTime
      settings: SourceProductName=MQTT
  port0_ci_ev_charge_remainingtimetofullsoc : speedgoatlib_mqtt/Client/MQTT Client Publish  ClientId=parClientId  ConnectionId=parConnectionId  Topic='port0/ci/ev/charge/remainingtimetofullsoc'  QoS=0 - at most once  Retain=on  Extended=on  SampleTime=parSampleTime
      settings: SourceProductName=MQTT
  port0_ci_ev_charge_resssoc : speedgoatlib_mqtt/Client/MQTT Client Publish  ClientId=parClientId  ConnectionId=parConnectionId  Topic='port0/ci/ev/charge/resssoc'  QoS=0 - at most once  Retain=on  Extended=on  SampleTime=parSampleTime
      settings: SourceProductName=MQTT
  port0_ci_ev_charge_targetcurrent : speedgoatlib_mqtt/Client/MQTT Client Publish  ClientId=parClientId  ConnectionId=parConnectionId  Topic='port0/ci/ev/charge/targetcurrent'  QoS=0 - at most once  Retain=on  Extended=on  SampleTime=parSampleTime
      settings: SourceProductName=MQTT
  port0_ci_ev_charge_targetvoltage : speedgoatlib_mqtt/Client/MQTT Client Publish  ClientId=parClientId  ConnectionId=parConnectionId  Topic='port0/ci/ev/charge/targetvoltage'  QoS=0 - at most once  Retain=on  Extended=on  SampleTime=parSampleTime
      settings: SourceProductName=MQTT
  to physical value format : MATLAB Function  TreatAsAtomicUnit=on
  to physical value format1 : MATLAB Function  TreatAsAtomicUnit=on
  to physical value format2 : MATLAB Function  TreatAsAtomicUnit=on
  to physical value format3 : MATLAB Function  TreatAsAtomicUnit=on
  wires:
  to physical value format3/1(multiplier) -> Function Caller7/1
  to physical value format3/2(value) -> Function Caller7/2
  Function Caller7/1 -> port0_ci_ev_charge_remainingtimetofullsoc/1
  Function Caller6/1 -> port0_ci_ev_charge_remainingtimetobulksoc/1
  to physical value format2/2(value) -> Function Caller6/2
  to physical value format2/1(multiplier) -> Function Caller6/1
  to physical value format1/1(multiplier) -> Function Caller5/1
  to physical value format1/2(value) -> Function Caller5/2
  Function Caller5/1 -> port0_ci_ev_charge_targetcurrent/1
  Function Caller13/1 -> port0_ci_ev_charge_targetvoltage/1
  to physical value format/2(value) -> Function Caller13/2
  to physical value format/1(multiplier) -> Function Caller13/1
  Data Type Conversion1/1 -> To String1/1
  remainingtimetofullsoc/1 -> to physical value format3/1(input)
  remainingtimetobulksoc/1 -> to physical value format2/1(input)
  chargingcomplete/1 -> To String4/1
  To String4/1 -> String to ASCII4/1
  String to ASCII4/1 -> port0_ci_ev_charge_chargingcomplete/1
  String to ASCII3/1 -> port0_ci_ev_charge_bulkchargingcomplete/1
  To String3/1 -> String to ASCII3/1
  bulkchargingcomplete/1 -> To String3/1
  resssoc/1 -> To String2/1
  To String2/1 -> String to ASCII2/1
  String to ASCII2/1 -> port0_ci_ev_charge_resssoc/1
  String to ASCII1/1 -> port0_ci_ev_charge_ready/1
  To String1/1 -> String to ASCII1/1
  chargeready/1 -> Data Type Conversion1/1
  chargingprofiletupleid/1 -> To String/1
  To String/1 -> String to ASCII/1
  String to ASCII/1 -> port0_ci_ev_charge_chargingprofiletupleid/1
  targetcurrent/1 -> to physical value format1/1(input)
  targetvoltage/1 -> to physical value format/1(input)
  Ground4/1 -> port0_ci_ev_charge_chargingprofiletupleid/3
  Constant4/1 -> port0_ci_ev_charge_chargingprofiletupleid/2
  Ground1/1 -> port0_ci_ev_charge_ready/3
  Constant1/1 -> port0_ci_ev_charge_ready/2
  Ground2/1 -> port0_ci_ev_charge_resssoc/3
  Constant2/1 -> port0_ci_ev_charge_resssoc/2
  Ground3/1 -> port0_ci_ev_charge_targetvoltage/3
  Constant3/1 -> port0_ci_ev_charge_targetvoltage/2
  Ground5/1 -> port0_ci_ev_charge_targetcurrent/3
  Constant5/1 -> port0_ci_ev_charge_targetcurrent/2
  Ground6/1 -> port0_ci_ev_charge_bulkchargingcomplete/3
  Constant6/1 -> port0_ci_ev_charge_bulkchargingcomplete/2
  Constant7/1 -> port0_ci_ev_charge_chargingcomplete/2
  Ground7/1 -> port0_ci_ev_charge_chargingcomplete/3
  Ground8/1 -> port0_ci_ev_charge_remainingtimetobulksoc/3
  Constant8/1 -> port0_ci_ev_charge_remainingtimetobulksoc/2
  Constant9/1 -> port0_ci_ev_charge_remainingtimetofullsoc/2
  Ground9/1 -> port0_ci_ev_charge_remainingtimetofullsoc/3
  To String5/1 -> String to ASCII5/1
  errorcode/1 -> To String5/1
  String to ASCII5/1 -> port0_ci_ev_charge_errorcode/1
  Ground10/1 -> port0_ci_ev_charge_errorcode/3
  Constant10/1 -> port0_ci_ev_charge_errorcode/2

== system speedgoatlib_evse/Blocks by Charge State/EV Charging Write /Enabled Subsystem1 ==
  readyToChargeState : Inport
  Enable : EnablePort
  Constant4 : Constant  Value=parEnReadyToChargeState  OutDataTypeStr=boolean
  Ground4 : Ground
  MQTT Client Publish : speedgoatlib_mqtt/Client/MQTT Client Publish  ClientId=parClientId  ConnectionId=parConnectionId  Topic='port0/ci/ev/charge/readytochargestate'  QoS=0 - at most once  Retain=on  Extended=on  SampleTime=parSampleTime
      settings: SourceProductName=MQTT
  String to ASCII : StringToASCII  OutputVectorSize=12
  To String : ToString
  wires:
  String to ASCII/1 -> MQTT Client Publish/1
  To String/1 -> String to ASCII/1
  readyToChargeState/1 -> To String/1
  Ground4/1 -> MQTT Client Publish/3
  Constant4/1 -> MQTT Client Publish/2
